simulink model "damper"  (R2021a)
settings: Solver=ode23t  StartTime=0.0  StopTime=10  MaxStep=0.08  RelTol=1e-3
values from neighbouring files (symbols this model uses):
  Fd = damper_R12_lo(:,1)'    [damperLUT.m]
  vel = damper_R12_lo(:,2)'    [damperLUT.m]
undefined symbols (not defined in the file or in its folder): coeff, length, X, Y, Z
libraries: sm_lib x11, nesl_utility x4
settings Model: Creator=Tarek  LastModifiedBy=Tarek

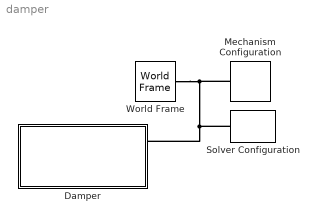
== system damper ==
  Damper : Subsystem
  Mechanism Configuration : sm_lib/Utilities/Mechanism Configuration  UniformGravity=Constant  GravityVector=[0 0 -9.80665]  GravityVectorUnits=m/s^2  GravityUnits=m/s^2  LinearizationDelta=0.001  JointModeTransitionNonlinearIterations=2
  Solver Configuration : nesl_utility/Solver Configuration  PhysicalDomain=network_engine_domain  SubClassName=solver  LeftPortType=input  RightPortType=generic  Tones=[]  Harmonics=[]  SimulateNoise=off  Profile=off  UseLocalSampling=off  EnableSwitchedLinearOptims=on  FrequencyDomain=off  UseCCode=off  RelTol=0.001  AbsTol=1e-06  MinStep=1e-09  ToWorkspace=off  RevertToSquareIcSolve=off  NumHomotopyIterations=100  PhasorMode=off  PhasorModeNumHarmonics=1  DoDC=off  ResidualTolerance=1e-09  UseLocalSolver=off  LocalSolverChoice=NE_BACKWARD_EULER_ADVANCER  LocalSolverSampleTime=0.001  DoFixedCost=off  MaxNonlinIter=3  MaxModeIter=2  ComputeImpulses=off  ImpulseIterations=2  LinearAlgebra=auto  EquationFormulation=NE_TIME_EF  DelaysMemoryBudget=1024  AutomaticFiltering=on  FilteringTimeConstant=0.001  PartitionStorageMethod=AS_NEEDED  PartitionMemoryBudget=1024  PartitionMethod=ROBUST
      settings: SourceProductBaseCode=PW,SS
  World Frame : sm_lib/Frames and Transforms/World Frame
  connections:
  World Frame/RConn1 -- Damper/RConn1 -- Solver Configuration/RConn1 -- Mechanism Configuration/RConn1

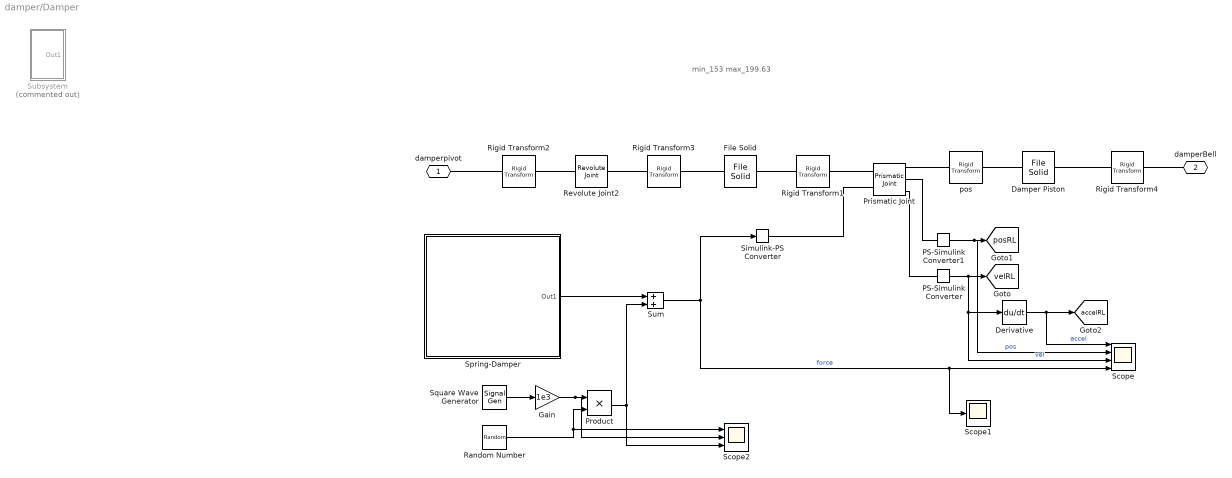
== system damper/Damper ==
  note: min_153
      | max_199.63
  Damper Piston : sm_lib/Body Elements/File Solid  ExtGeomFileName=C:\Users\Tarek\Documents\GitHub\SimulinkMBS\CADs\Suspension\Damper_Piston.stl  UnitType=Custom  ExtGeomFileUnits=mm  StepReaderType=HEX  ExportConvexHullGeometry=off  InertiaType=CalculateFromGeometry  Mass=394*.25  MassUnits=g  CenterOfMass=[0 0 0]  CenterOfMassUnits=m  MomentsOfInertia=[1 1 1]  MomentsOfInertiaUnits=kg*m^2  ProductsOfInertia=[0 0 0]  ProductsOfInertiaUnits=kg*m^2  BasedOnType=Mass  Density=1000  DensityUnits=kg/m^3  DoExposeReferenceFrame=on  SerializedFrames=<Frames><Frame><Id>Frame1</Id><Value><Name>F1</Name><Origin><Source>ReferenceFrame</Source><FeatureName></FeatureName></Origin><PrimaryAxis><DefinedDirection>+Z</DefinedDirection><Source>ReferenceFrame</Source><SourceDirection>+Z</SourceDirection><FeatureName></FeatureName></PrimaryAxis><SecondaryAxis><DefinedDirection>+X</DefinedDirection><Source>ReferenceFrame</Source><SourceDirection>+X</SourceDirection><FeatureName></FeatureName></SecondaryAxis></Value></Frame></Frames>  GraphicType=FromGeometry  MarkerShape=Sphere  MarkerSize=10  GraphicVisPropType=SimpleVisualProperties  GraphicDiffuseColor=[0.5 0.5 0.5]  GraphicSpecularColor=[0.5 0.5 0.5 1.0]  GraphicAmbientColor=[0.15 0.15 0.15 1.0]  GraphicEmissiveColor=[0.0 0.0 0.0 1.0]  GraphicShininess=75  GraphicOpacity=1.0
  Derivative : Derivative
  File Solid : sm_lib/Body Elements/File Solid  ExtGeomFileName=C:\Users\Tarek\Documents\GitHub\SimulinkMBS\CADs\Suspension\Damper_Base.stl  UnitType=Custom  ExtGeomFileUnits=mm  StepReaderType=HEX  ExportConvexHullGeometry=off  InertiaType=CalculateFromGeometry  Mass=394*.75  MassUnits=g  CenterOfMass=[0 0 0]  CenterOfMassUnits=m  MomentsOfInertia=[1 1 1]  MomentsOfInertiaUnits=kg*m^2  ProductsOfInertia=[0 0 0]  ProductsOfInertiaUnits=kg*m^2  BasedOnType=Mass  Density=1000  DensityUnits=kg/m^3  DoExposeReferenceFrame=on  SerializedFrames=<Frames><Frame><Id>Frame1</Id><Value><Name>F1</Name><Origin><Source>ReferenceFrame</Source><FeatureName></FeatureName></Origin><PrimaryAxis><DefinedDirection>+Z</DefinedDirection><Source>ReferenceFrame</Source><SourceDirection>+Z</SourceDirection><FeatureName></FeatureName></PrimaryAxis><SecondaryAxis><DefinedDirection>+X</DefinedDirection><Source>ReferenceFrame</Source><SourceDirection>+X</SourceDirection><FeatureName></FeatureName></SecondaryAxis></Value></Frame></Frames>  GraphicType=FromGeometry  MarkerShape=Sphere  MarkerSize=10  GraphicVisPropType=SimpleVisualProperties  GraphicDiffuseColor=[0.5 0.5 0.5]  GraphicSpecularColor=[0.5 0.5 0.5 1.0]  GraphicAmbientColor=[0.15 0.15 0.15 1.0]  GraphicEmissiveColor=[0.0 0.0 0.0 1.0]  GraphicShininess=75  GraphicOpacity=1.0
  Gain : Gain  Gain=1e3
  PS-Simulink Converter : nesl_utility/PS-Simulink Converter  PhysicalDomain=network_engine_domain  SubClassName=ps_output  LeftPortType=input  RightPortType=output  PseudoPeriodic=off  Frequencies=[]  Unit=inherit  AffineConversion=off
      settings: SourceProductBaseCode=PW,SS
  PS-Simulink Converter1 : nesl_utility/PS-Simulink Converter  PhysicalDomain=network_engine_domain  SubClassName=ps_output  LeftPortType=input  RightPortType=output  PseudoPeriodic=off  Frequencies=[]  Unit=inherit  AffineConversion=off
      settings: SourceProductBaseCode=PW,SS
  Prismatic Joint : sm_lib/Joints/Prismatic Joint  JointMode=Normal  SenseConstraintForce=off  SenseConstraintForceX=off  SenseConstraintForceY=off  SenseConstraintForceZ=off  SenseConstraintTorque=off  SenseConstraintTorqueX=off  SenseConstraintTorqueY=off  SenseConstraintTorqueZ=off  SenseTotalForce=off  SenseTotalForceX=off  SenseTotalForceY=off  SenseTotalForceZ=off  SenseTotalTorque=off  SenseTotalTorqueX=off  SenseTotalTorqueY=off  SenseTotalTorqueZ=off  CompositeWrenchDir=FollowerOnBase  CompositeWrenchFrame=BaseFrame  EquilibriumPosition=0  EquilibriumPositionUnits=m  SpringStiffness=0  SpringStiffnessUnits=N/m  DampingCoefficient=0  DampingCoefficientUnits=N/(m/s)  TorqueActuationMode=InputTorque  MotionActuationMode=ComputedMotion  SensePosition=on  SenseVelocity=on  SenseAcceleration=off  SenseTorqueForce=off  SenseLowerLimitTorqueForce=off  SenseUpperLimitTorqueForce=off  LowerLimitSpecify=on  LowerLimitBound=length.stroke.min  LowerLimitBoundUnits=mm  LowerLimitStiffness=1e6  LowerLimitStiffnessUnits=N/m  LowerLimitDamping=1e3  LowerLimitDampingUnits=N/(m/s)  LowerLimitTransitionRegionWidth=1e-4  LowerLimitTransitionRegionWidthUnits=m  UpperLimitSpecify=on  UpperLimitBound=length.stroke.max  UpperLimitBoundUnits=mm  UpperLimitStiffness=1e6  UpperLimitStiffnessUnits=N/m  UpperLimitDamping=1e3  UpperLimitDampingUnits=N/(m/s)  UpperLimitTransitionRegionWidth=1e-4  UpperLimitTransitionRegionWidthUnits=m  PositionTargetSpecify=off  PositionTargetPriority=High  PositionTargetValue=0  PositionTargetValueUnits=m  VelocityTargetSpecify=off  VelocityTargetPriority=High  VelocityTargetValue=0  VelocityTargetValueUnits=m/s
  Product : Product
  Random Number : RandomNumber  Mean=-1  SampleTime=.5
  Revolute Joint2 : sm_lib/Joints/Revolute Joint  JointMode=Normal  SenseConstraintForce=off  SenseConstraintForceX=off  SenseConstraintForceY=off  SenseConstraintForceZ=off  SenseConstraintTorque=off  SenseConstraintTorqueX=off  SenseConstraintTorqueY=off  SenseConstraintTorqueZ=off  SenseTotalForce=off  SenseTotalForceX=off  SenseTotalForceY=off  SenseTotalForceZ=off  SenseTotalTorque=off  SenseTotalTorqueX=off  SenseTotalTorqueY=off  SenseTotalTorqueZ=off  CompositeWrenchDir=FollowerOnBase  CompositeWrenchFrame=BaseFrame  EquilibriumPosition=0  EquilibriumPositionUnits=deg  SpringStiffness=0  SpringStiffnessUnits=N*m/deg  DampingCoefficient=0  DampingCoefficientUnits=N*m/(deg/s)  TorqueActuationMode=NoTorque  MotionActuationMode=ComputedMotion  SensePosition=off  SenseVelocity=off  SenseAcceleration=off  SenseTorqueForce=off  SenseLowerLimitTorqueForce=off  SenseUpperLimitTorqueForce=off  LowerLimitSpecify=off  LowerLimitBound=-90  LowerLimitBoundUnits=deg  LowerLimitStiffness=1e4  LowerLimitStiffnessUnits=N*m/deg  LowerLimitDamping=10  LowerLimitDampingUnits=N*m/(deg/s)  LowerLimitTransitionRegionWidth=0.1  LowerLimitTransitionRegionWidthUnits=deg  UpperLimitSpecify=off  UpperLimitBound=90  UpperLimitBoundUnits=deg  UpperLimitStiffness=1e4  UpperLimitStiffnessUnits=N*m/deg  UpperLimitDamping=10  UpperLimitDampingUnits=N*m/(deg/s)  UpperLimitTransitionRegionWidth=0.1  UpperLimitTransitionRegionWidthUnits=deg  PositionTargetSpecify=off  PositionTargetPriority=High  PositionTargetValue=0  PositionTargetValueUnits=deg  VelocityTargetSpecify=off  VelocityTargetPriority=High  VelocityTargetValue=0  VelocityTargetValueUnits=deg/s
  Rigid Transform1 : sm_lib/Frames and Transforms/Rigid Transform  TranslationMethod=None  TranslationStandardOffset=50  TranslationLengthUnit=mm  TranslationStandardAxis=-Y  TranslationCartesianOffset=[0 0 0]  TranslationROffset=0  TranslationROffsetUnits=m  TranslationZOffset=0  TranslationZOffsetUnits=m  TranslationThetaOffset=0  TranslationThetaOffsetUnits=deg  RotationMethod=StandardAxis  RotationAngleUnits=deg  RotationStandardAxis=+X  RotationAngle=90  RotationArbitraryAxis=[0 0 1]  FollAlignAxisA=+Z  BaseAlignAxisA=+Y  FollAlignAxisB=+Y  BaseAlignAxisB=+Z  RotationSequenceAxes=FollowerAxes  RotationSequence=XYX  RotationSequenceAngles=[0 0 0]  RotationSequenceAnglesUnits=deg  RotationMatrix=[1 0 0; 0 1 0; 0 0 1]
  Rigid Transform2 : sm_lib/Frames and Transforms/Rigid Transform  TranslationMethod=None  TranslationStandardOffset=0  TranslationLengthUnit=m  TranslationStandardAxis=+Z  TranslationCartesianOffset=[0 0 0]  TranslationROffset=0  TranslationROffsetUnits=m  TranslationZOffset=0  TranslationZOffsetUnits=m  TranslationThetaOffset=0  TranslationThetaOffsetUnits=deg  RotationMethod=RotationSequence  RotationAngleUnits=deg  RotationStandardAxis=+Z  RotationAngle=0.0  RotationArbitraryAxis=[0 0 1]  FollAlignAxisA=+X  BaseAlignAxisA=+Y  FollAlignAxisB=+Y  BaseAlignAxisB=+Z  RotationSequenceAxes=FollowerAxes  RotationSequence=XYX  RotationSequenceAngles=[0 180 0]  RotationSequenceAnglesUnits=deg  RotationMatrix=[1 0 0; 0 1 0; 0 0 1]
  Rigid Transform3 : sm_lib/Frames and Transforms/Rigid Transform  TranslationMethod=None  TranslationStandardOffset=110/2  TranslationLengthUnit=mm  TranslationStandardAxis=-Z  TranslationCartesianOffset=[0 0 0]  TranslationROffset=0  TranslationROffsetUnits=m  TranslationZOffset=0  TranslationZOffsetUnits=m  TranslationThetaOffset=0  TranslationThetaOffsetUnits=deg  RotationMethod=RotationSequence  RotationAngleUnits=deg  RotationStandardAxis=-Y  RotationAngle=90  RotationArbitraryAxis=[0 0 1]  FollAlignAxisA=+Y  BaseAlignAxisA=+Y  FollAlignAxisB=+X  BaseAlignAxisB=+X  RotationSequenceAxes=FollowerAxes  RotationSequence=ZXY  RotationSequenceAngles=[-90 90 0]  RotationSequenceAnglesUnits=deg  RotationMatrix=[1 0 0; 0 1 0; 0 0 1]
  Rigid Transform4 : sm_lib/Frames and Transforms/Rigid Transform  TranslationMethod=None  TranslationStandardOffset=170/2  TranslationLengthUnit=mm  TranslationStandardAxis=+Z  TranslationCartesianOffset=[0 0 0]  TranslationROffset=0  TranslationROffsetUnits=m  TranslationZOffset=0  TranslationZOffsetUnits=m  TranslationThetaOffset=0  TranslationThetaOffsetUnits=deg  RotationMethod=RotationSequence  RotationAngleUnits=deg  RotationStandardAxis=-Y  RotationAngle=90  RotationArbitraryAxis=[0 0 1]  FollAlignAxisA=+X  BaseAlignAxisA=+Y  FollAlignAxisB=+Y  BaseAlignAxisB=+Z  RotationSequenceAxes=FollowerAxes  RotationSequence=ZXY  RotationSequenceAngles=[-90 90 0]  RotationSequenceAnglesUnits=deg  RotationMatrix=[1 0 0; 0 1 0; 0 0 1]
  Scope : Scope  NumInputPorts=4
  Scope1 : Scope
  Scope2 : Scope  NumInputPorts=3
  Simulink-PS Converter : nesl_utility/Simulink-PS Converter  PhysicalDomain=network_engine_domain  SubClassName=ps_input  LeftPortType=input  RightPortType=output  PseudoPeriodic=off  Frequencies=[]  NoiseDistribution=none  NoiseParameters=[]  Unit=1  AffineConversion=off  FilteringAndDerivatives=provide  SimscapeFilterOrder=1  InputFilterTimeConstant=0.001  UdotUserProvided=0
      settings: SourceProductBaseCode=PW,SS
  Spring-Damper : Subsystem
  Square Wave Generator : SignalGenerator
  Subsystem : Subsystem  Commented=on
  Sum : Sum
  pos : sm_lib/Frames and Transforms/Rigid Transform  TranslationMethod=StandardAxis  TranslationStandardOffset=length.stroke.midref  TranslationLengthUnit=mm  TranslationStandardAxis=+Z  TranslationCartesianOffset=[ 0.00000000, -175.08521427, 8.82725061 ]  TranslationROffset=0  TranslationROffsetUnits=m  TranslationZOffset=0  TranslationZOffsetUnits=m  TranslationThetaOffset=0  TranslationThetaOffsetUnits=deg  RotationMethod=StandardAxis  RotationAngleUnits=deg  RotationStandardAxis=-X  RotationAngle=90  RotationArbitraryAxis=[0 0 1]  FollAlignAxisA=+X  BaseAlignAxisA=+Y  FollAlignAxisB=+Y  BaseAlignAxisB=+Z  RotationSequenceAxes=FollowerAxes  RotationSequence=XYX  RotationSequenceAngles=[0 0 0]  RotationSequenceAnglesUnits=deg  RotationMatrix=[1 0 0; 0 1 0; 0 0 1]
  damperpivot : PMIOPort  Side=Right
  damperBell : PMIOPort  Port=2  Side=Right
  tag scope: accelRL=global, posRL=global, velRL=global
  wires:
  PS-Simulink Converter/1 -> Derivative/1, Scope/3, [velRL]  "vel"
  PS-Simulink Converter1/1 -> Scope/2, [posRL]  "pos"
  Derivative/1 -> Scope/1, [accelRL]  "accel"
  Sum/1 -> Scope1/1, Scope/4, Simulink-PS Converter/1  "force"
  Spring-Damper/1(Out1) -> Sum/1
  Square Wave Generator/1 -> Gain/1
  Gain/1 -> Scope2/2, Product/1
  Product/1 -> Scope2/3, Sum/2
  Random Number/1 -> Product/2, Scope2/1
  connections:
  File Solid/LConn1 -- Rigid Transform1/LConn1
  Prismatic Joint/RConn1 -- pos/LConn1
  Damper Piston/LConn1 -- Rigid Transform4/LConn1
  pos/RConn1 -- Damper Piston/RConn1
  Rigid Transform2/LConn1 -- Revolute Joint2/LConn1
  Rigid Transform4/RConn1 -- damperBell/RConn1
  Revolute Joint2/RConn1 -- Rigid Transform3/RConn1
  Rigid Transform3/LConn1 -- File Solid/RConn1
  Rigid Transform1/RConn1 -- Prismatic Joint/LConn1
  damperpivot/RConn1 -- Rigid Transform2/RConn1
  PS-Simulink Converter/LConn1 -- Prismatic Joint/RConn3
  PS-Simulink Converter1/LConn1 -- Prismatic Joint/RConn2
  Prismatic Joint/LConn2 -- Simulink-PS Converter/RConn1

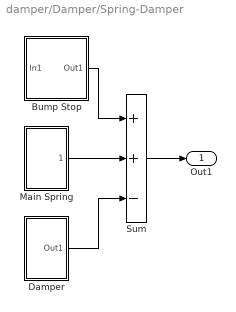
== system damper/Damper/Spring-Damper ==
  Bump Stop : Subsystem
  Damper : Subsystem
  Main Spring : Subsystem
  Sum : Sum  Inputs=++-
  Out1 : Outport
  wires:
  Sum/1 -> Out1/1
  Main Spring/1(forces) -> Sum/2
  Damper/1(Out1) -> Sum/3
  Bump Stop/1(Out1) -> Sum/1

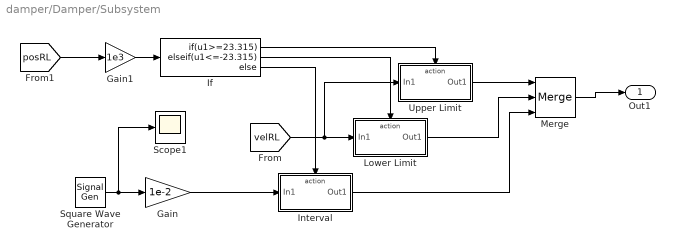
== system damper/Damper/Subsystem ==
  Gain : Gain  Gain=1e-2
  Gain1 : Gain  Gain=1e3
  If : If  IfExpression=u1>=23.315  ElseIfExpressions=u1<=-23.315
  Interval : Subsystem  TreatAsAtomicUnit=on
  Lower Limit : Subsystem  TreatAsAtomicUnit=on
  Merge : Merge  Inputs=3
  Scope1 : Scope
  Square Wave Generator : SignalGenerator  WaveForm=square  Amplitude=-1  Frequency=0.5  Units=rad/sec
  Upper Limit : Subsystem  TreatAsAtomicUnit=on
  Out1 : Outport
  wires:
  Gain/1 -> Interval/1(In1)
  If/3 -> Interval/Action
  Gain1/1 -> If/1
  Lower Limit/1(Out1) -> Merge/2
  [posRL] -> Gain1/1
  Upper Limit/1(Out1) -> Merge/1
  Interval/1(Out1) -> Merge/3
  If/1 -> Upper Limit/Action
  Square Wave Generator/1 -> Scope1/1, Gain/1
  If/2 -> Lower Limit/Action
  [velRL] -> Upper Limit/1(In1), Lower Limit/1(In1)
  Merge/1 -> Out1/1

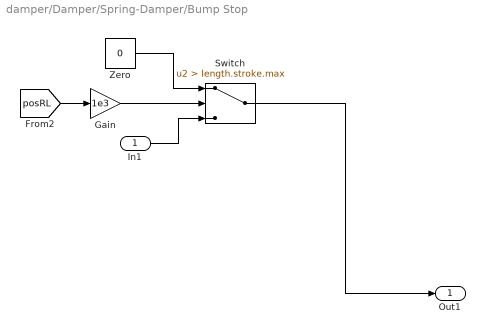
== system damper/Damper/Spring-Damper/Bump Stop ==
  In1 : Inport
  Gain : Gain  Gain=1e3
  Switch : Switch  Criteria=u2 > Threshold  Threshold=length.stroke.max
  Zero : Constant  Value=0  OutDataTypeStr=Inherit: Inherit via back propagation
  Out1 : Outport
  wires:
  Gain/1 -> Switch/2
  In1/1 -> Switch/3
  Switch/1 -> Out1/1
  [posRL] -> Gain/1
  Zero/1 -> Switch/1

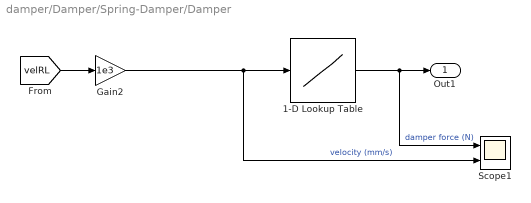
== system damper/Damper/Spring-Damper/Damper ==
  1-D Lookup Table : Lookup_n-D  NumberOfTableDimensions=1  BreakpointsForDimension1=Fd  Table=vel  InternalRulePriority=Speed  RndMeth=Simplest  InputSameDT=on
  Gain2 : Gain  Gain=1e3
  Scope1 : Scope  NumInputPorts=2
  Out1 : Outport
  wires:
  [velRL] -> Gain2/1
  Gain2/1 -> Scope1/2, 1-D Lookup Table/1  "velocity (mm/s)"
  1-D Lookup Table/1 -> Scope1/1, Out1/1  "damper force (N)"

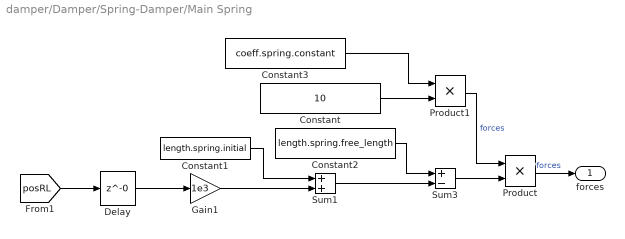
== system damper/Damper/Spring-Damper/Main Spring ==
  Constant : Constant  Value=10
  Constant1 : Constant  Value=length.spring.initial  VectorParams1D=off
  Constant2 : Constant  Value=length.spring.free_length  VectorParams1D=off
  Constant3 : Constant  Value=coeff.spring.constant  VectorParams1D=off
  Delay : Delay  DelayLength=0
  Gain1 : Gain  Gain=1e3
  Product : Product
  Product1 : Product
  Sum1 : Sum
  Sum3 : Sum  Inputs=+-
  forces : Outport
  wires:
  Gain1/1 -> Sum1/2
  [posRL] -> Delay/1
  Product1/1 -> Product/1  "forces"
  Constant1/1 -> Sum1/1
  Product/1 -> forces/1  "forces"
  Constant3/1 -> Product1/1
  Sum1/1 -> Sum3/2
  Constant/1 -> Product1/2
  Constant2/1 -> Sum3/1
  Sum3/1 -> Product/2
  Delay/1 -> Gain1/1

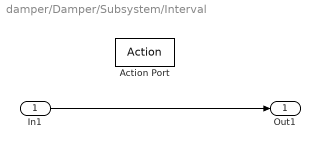
== system damper/Damper/Subsystem/Interval ==
  In1 : Inport
  Action Port : ActionPort  ActionPortLabel=else
  Out1 : Outport
  wires:
  In1/1 -> Out1/1

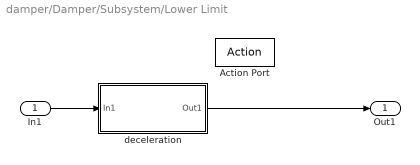
== system damper/Damper/Subsystem/Lower Limit ==
  In1 : Inport
  Action Port : ActionPort  ActionPortLabel=elseif(u1<=-23.315)
  deceleration : Subsystem
  Out1 : Outport
  wires:
  In1/1 -> deceleration/1(In1)
  deceleration/1(Out1) -> Out1/1

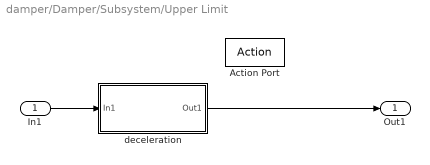
== system damper/Damper/Subsystem/Upper Limit ==
  In1 : Inport
  Action Port : ActionPort  ActionPortLabel=if(u1>=23.315)
  deceleration : Subsystem
  Out1 : Outport
  wires:
  In1/1 -> deceleration/1(In1)
  deceleration/1(Out1) -> Out1/1

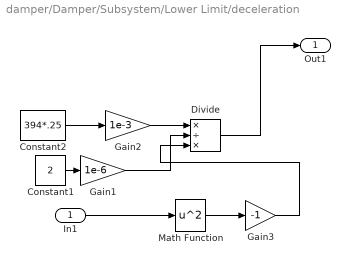
== system damper/Damper/Subsystem/Lower Limit/deceleration ==
  In1 : Inport
  Constant1 : Constant  Value=2
  Constant2 : Constant  Value=394*.25
  Divide : Product  Inputs=*/*
  Gain1 : Gain  Gain=1e-6
  Gain2 : Gain  Gain=1e-3
  Gain3 : Gain  Gain=-1
  Math Function : Math  Operator=square  SaturateOnIntegerOverflow=on
  Out1 : Outport
  wires:
  In1/1 -> Math Function/1
  Math Function/1 -> Gain3/1
  Gain3/1 -> Divide/3
  Constant2/1 -> Gain2/1
  Gain2/1 -> Divide/1
  Divide/1 -> Out1/1
  Gain1/1 -> Divide/2
  Constant1/1 -> Gain1/1

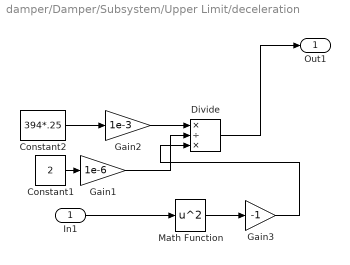
== system damper/Damper/Subsystem/Upper Limit/deceleration ==
  In1 : Inport
  Constant1 : Constant  Value=2
  Constant2 : Constant  Value=394*.25
  Divide : Product  Inputs=*/*
  Gain1 : Gain  Gain=1e-6
  Gain2 : Gain  Gain=1e-3
  Gain3 : Gain  Gain=-1
  Math Function : Math  Operator=square  SaturateOnIntegerOverflow=on
  Out1 : Outport
  wires:
  In1/1 -> Math Function/1
  Math Function/1 -> Gain3/1
  Gain3/1 -> Divide/3
  Constant2/1 -> Gain2/1
  Gain2/1 -> Divide/1
  Divide/1 -> Out1/1
  Gain1/1 -> Divide/2
  Constant1/1 -> Gain1/1
